simulink model "bmw_drive_force"  (R2022b)
settings: Solver=ode45  StartTime=0.0  StopTime=15  RelTol=1e-3  EnableMultiTasking=on
PreLoadFcn:
  | % Parameters
  | load gear_data;
  | FDR = 3.23;
  | AvgEngTorque = 222;
  | Loss = 0.8;
  | r_tire = 1.030;
settings Model: Creator=jrivitus  LastModifiedBy=bensweet
settings SolverCC: AlgebraicLoopSolver=TrustRegion
settings DataIOCC: ExternalInput=[t, gear]  LimitDataPoints=on  LoadExternalInput=on  SaveFormat=Array  ReturnWorkspaceOutputs=off
settings OptimizationCC: ExpressionDepthLimit=2147483647  LifeSpan=inf
settings DebuggingCC: UnconnectedInputMsg=warning  UnconnectedOutputMsg=warning  UnconnectedLineMsg=warning  PregeneratedLibrarySubsystemCodeDiagnostic=none  SFMachineParentedDataDiag=warning
settings HardwareCC: ProdBitPerPointer=32  ProdBitPerSizeT=32  ProdBitPerPtrDiffT=32  ProdLargestAtomicFloat=None  ProdIntDivRoundTo=Undefined  ProdEndianess=Unspecified  ProdWordSize=32  ProdHWDeviceType=32-bit Generic
settings ModelReferenceCC: EnableRefExpFcnMdlSchedulingChecks=on  PropagateSignalLabelsOutOfModel=off
settings SFSimCC: SimUseLocalCustomCode=off
settings RTWCC: RTWUseLocalCustomCode=off  DLArmComputeVersion=19.05
settings CodeAppCC: StateflowObjectComments=on
settings GRTTargetCC: TargetLangStandard=C89/C90 (ANSI)  CombineOutputUpdateFcns=off  GRTInterface=on
settings ConfigComp: CovMetricSettings=dw  CovSaveCumulativeToWorkspaceVar=on  CovSaveSingleToWorkspaceVar=on  CovExternalEMLEnable=off  CovSFcnEnable=off

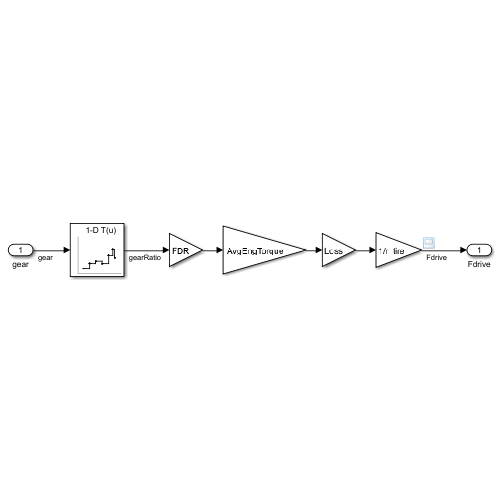
[thumbnail: Simulink's stored preview of the top-level diagram]
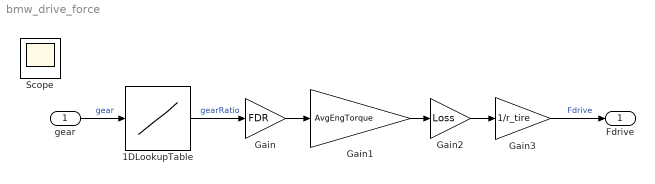
== system bmw_drive_force ==
  gear : Inport
  1DLookupTable : Lookup_n-D  NumberOfTableDimensions=1  BreakpointsForDimension1=[1:5]  Table=[4.21 2.49 1.66 1.24 1.00]  InterpMethod=Flat  ExtrapMethod=Clip  RndMeth=Simplest
  Gain : Gain  Gain=FDR
  Gain1 : Gain  Gain=AvgEngTorque
  Gain2 : Gain  Gain=Loss
  Gain3 : Gain  Gain=1/r_tire
  Fdrive : Outport  VectorParamsAs1DForOutWhenUnconnected=off
  Scope : Scope
  wires:
  gear/1 -> 1DLookupTable/1  "gear"
  1DLookupTable/1 -> Gain/1  "gearRatio"
  Gain/1 -> Gain1/1
  Gain1/1 -> Gain2/1
  Gain2/1 -> Gain3/1
  Gain3/1 -> Fdrive/1  "Fdrive"
